simulink model "Teleoperation_no_voltage_no_force_control"  (R2020a)
settings: Solver=VariableStepAuto  StartTime=0.0  StopTime=10  RelTol=1e-3
values from neighbouring files (symbols this model uses):
  B = 1/k_m    (= 0.0517063081696)    [Teleop_parameters.m]    (also in base.mat; base_no_attrito.mat = 0; ci_siamo.mat; force_control.mat)
  Be = 5    [Teleop_parameters.m]    (also in base.mat = 0.5; base_no_attrito.mat = 0.5; ci_siamo.mat; force_control.mat = 0.5)
  Bh = 0.02    [Teleop_parameters.m]    (also in base.mat; base_no_attrito.mat; ci_siamo.mat; force_control.mat)
  Fc_h = 5    [Teleop_parameters.m]    (also in base.mat; base_no_attrito.mat; ci_siamo.mat; force_control.mat)
  J = tau_m/k_m    (= 0.0629265770424)    [Teleop_parameters.m]    (also in base.mat; base_no_attrito.mat; ci_siamo.mat; force_control.mat)
  Jh = 0.02    [Teleop_parameters.m]    (also in base.mat; base_no_attrito.mat; ci_siamo.mat; force_control.mat)
  Kd_h = 0.5    [Teleop_parameters.m]    (also in base.mat = 1; base_no_attrito.mat = 1; ci_siamo.mat = 10; force_control.mat = 1)
  Kd_m = 0.005    [Teleop_parameters.m]    (also in base.mat = 1; base_no_attrito.mat = 1; ci_siamo.mat; force_control.mat = 1)
  Kd_s = 0.5    [Teleop_parameters.m]    (also in base.mat = 1; base_no_attrito.mat = 1; ci_siamo.mat; force_control.mat = 1)
  Ke = 10    [Teleop_parameters.m]    (also in base.mat; base_no_attrito.mat; ci_siamo.mat; force_control.mat)
  Kp_h = 1.2    [Teleop_parameters.m]    (also in base.mat; base_no_attrito.mat; ci_siamo.mat = 10; force_control.mat)
  Kp_m = 0.01    [Teleop_parameters.m]    (also in base.mat = 1; base_no_attrito.mat = 1; ci_siamo.mat; force_control.mat = 1)
  Kp_s = 1    [Teleop_parameters.m]    (also in base.mat; base_no_attrito.mat; ci_siamo.mat; force_control.mat)
  qe = 1.2    [Teleop_parameters.m]    (also in base.mat = 5; base_no_attrito.mat = 5; ci_siamo.mat = 0.5; force_control.mat = 5)
settings Model: Creator=kriato  LastModifiedBy=giovanni

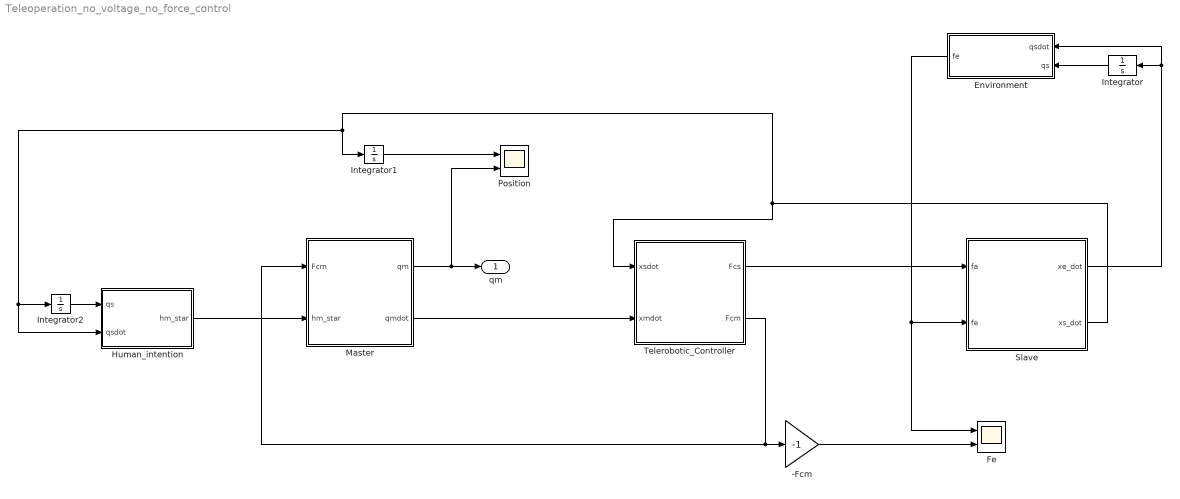
== system Teleoperation_no_voltage_no_force_control ==
  -Fcm : Gain  Gain=-1
  Environment : Subsystem
  Fe : Scope  NumInputPorts=2
  Human_intention : Subsystem
  Integrator : Integrator
  Integrator1 : Integrator
  Integrator2 : Integrator
  Master : Subsystem
  Position : Scope  NumInputPorts=2
  Slave : Subsystem
  Telerobotic_Controller : Subsystem
  qm : Outport
  wires:
  Master/2(qmdot) -> Telerobotic_Controller/2(xmdot)
  Slave/2(xs_dot) -> Human_intention/2(qsdot), Integrator2/1, Integrator1/1, Telerobotic_Controller/1(xsdot)
  Environment/1(fe) -> Slave/2(fe), Fe/1
  Master/1(qm) -> Position/2, qm/1
  Slave/1(xe_dot) -> Environment/1(qsdot), Integrator/1
  -Fcm/1 -> Fe/2
  Human_intention/1(hm_star) -> Master/2(hm_star)
  Telerobotic_Controller/1(Fcs) -> Slave/1(fa)
  Integrator/1 -> Environment/2(qs)
  Telerobotic_Controller/2(Fcm) -> Master/1(Fcm), -Fcm/1
  Integrator1/1 -> Position/1
  Integrator2/1 -> Human_intention/1(qs)

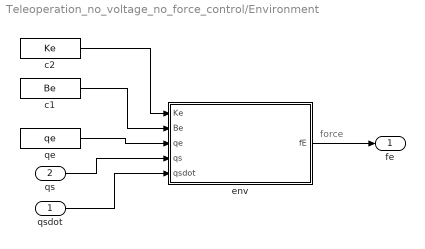
== system Teleoperation_no_voltage_no_force_control/Environment ==
  note: force
  qsdot : Inport
  qs : Inport  Port=2
  c1 : Constant  Value=Be  SampleTime=0
  c2 : Constant  Value=Ke  SampleTime=0
  env : MATLAB Function  TreatAsAtomicUnit=on
  qe : Constant  Value=qe  SampleTime=0
  fe : Outport  VectorParamsAs1DForOutWhenUnconnected=off
  wires:
  qe/1 -> env/3(qe)
  c1/1 -> env/2(Be)
  c2/1 -> env/1(Ke)
  qs/1 -> env/4(qs)
  qsdot/1 -> env/5(qsdot)
  env/1(fE) -> fe/1

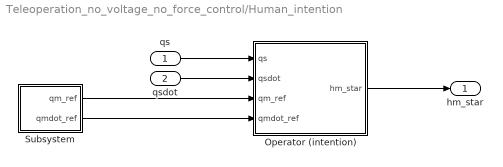
== system Teleoperation_no_voltage_no_force_control/Human_intention ==
  qs : Inport
  qsdot : Inport  Port=2
  Operator (intention) : Subsystem
  Subsystem : Subsystem
  hm_star : Outport
  wires:
  Subsystem/1(qm_ref) -> Operator (intention)/3(qm_ref)
  Subsystem/2(qmdot_ref) -> Operator (intention)/4(qmdot_ref)
  Operator (intention)/1(hm_star) -> hm_star/1
  qs/1 -> Operator (intention)/1(qs)
  qsdot/1 -> Operator (intention)/2(qsdot)

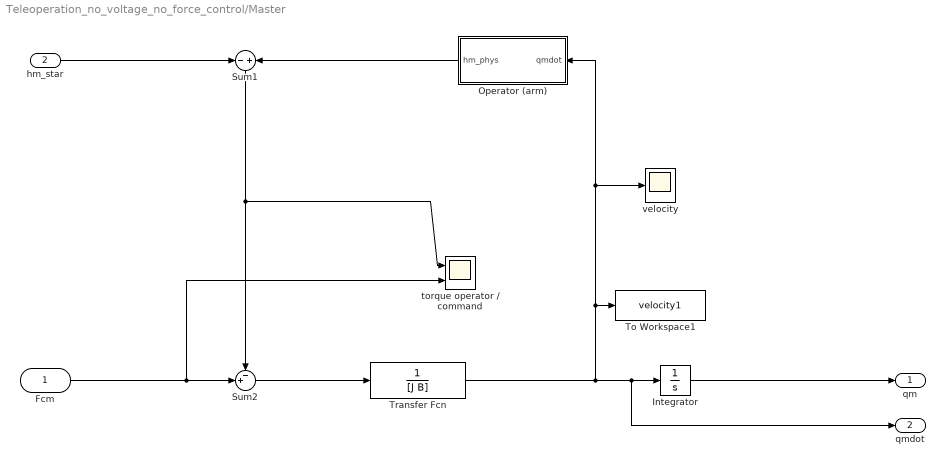
== system Teleoperation_no_voltage_no_force_control/Master ==
  Fcm : Inport
  hm_star : Inport  Port=2
  Integrator : Integrator
  Operator (arm) : Subsystem
  Sum1 : Sum  Inputs=-+
  Sum2 : Sum  Inputs=-+|
  To Workspace1 : ToWorkspace  VariableName=velocity1  SaveFormat=Timeseries  SampleTime=-1
  Transfer Fcn : TransferFcn  Denominator=[J B]
  torque operator / command : Scope  NumInputPorts=2
  velocity : Scope
  qm : Outport
  qmdot : Outport  Port=2
  wires:
  Integrator/1 -> qm/1
  Operator (arm)/1(hm_phys) -> Sum1/2
  Sum1/1 -> Sum2/1, torque operator / command/1
  Fcm/1 -> torque operator / command/2, Sum2/2
  Transfer Fcn/1 -> Operator (arm)/1(qmdot), velocity/1, To Workspace1/1, qmdot/1, Integrator/1
  hm_star/1 -> Sum1/1
  Sum2/1 -> Transfer Fcn/1

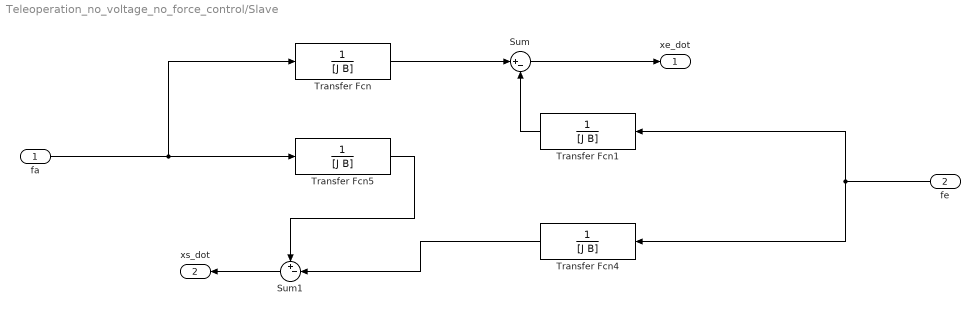
== system Teleoperation_no_voltage_no_force_control/Slave ==
  fa : Inport
  fe : Inport  Port=2
  Sum : Sum  Inputs=|+-
  Sum1 : Sum  Inputs=+-|
  Transfer Fcn{,1,4..5} (4 alike) : TransferFcn  Denominator=[J B]
  xe_dot : Outport
  xs_dot : Outport  Port=2
  wires:
  fa/1 -> Transfer Fcn5/1, Transfer Fcn/1
  Transfer Fcn/1 -> Sum/1
  Sum/1 -> xe_dot/1
  Transfer Fcn1/1 -> Sum/2
  Transfer Fcn4/1 -> Sum1/2
  Transfer Fcn5/1 -> Sum1/1
  Sum1/1 -> xs_dot/1
  fe/1 -> Transfer Fcn4/1, Transfer Fcn1/1

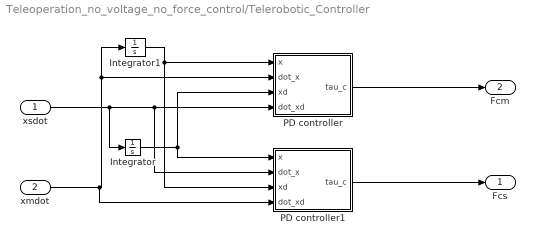
== system Teleoperation_no_voltage_no_force_control/Telerobotic_Controller ==
  xsdot : Inport
  xmdot : Inport  Port=2
  Integrator : Integrator
  Integrator1 : Integrator
  PD controller : Subsystem
  PD controller1 : Subsystem
  Fcs : Outport
  Fcm : Outport  Port=2
  wires:
  Integrator/1 -> PD controller1/1(x), PD controller/3(xd)
  Integrator1/1 -> PD controller1/3(xd), PD controller/1(x)
  xsdot/1 -> PD controller1/2(dot_x), PD controller/4(dot_xd), Integrator/1
  xmdot/1 -> PD controller1/4(dot_xd), PD controller/2(dot_x), Integrator1/1
  PD controller/1(tau_c) -> Fcm/1
  PD controller1/1(tau_c) -> Fcs/1

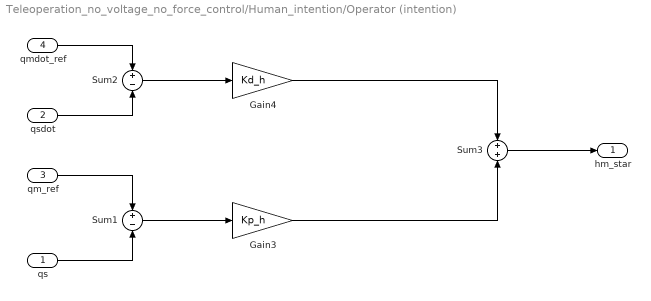
== system Teleoperation_no_voltage_no_force_control/Human_intention/Operator (intention) ==
  qs : Inport
  qsdot : Inport  Port=2
  qm_ref : Inport  Port=3
  qmdot_ref : Inport  Port=4
  Gain3 : Gain  Gain=Kp_h
  Gain4 : Gain  Gain=Kd_h
  Sum1 : Sum  Inputs=+|-
  Sum2 : Sum  Inputs=+|-
  Sum3 : Sum  Inputs=+|+
  hm_star : Outport  VectorParamsAs1DForOutWhenUnconnected=off
  wires:
  qs/1 -> Sum1/2
  qm_ref/1 -> Sum1/1
  qmdot_ref/1 -> Sum2/1
  Sum1/1 -> Gain3/1
  qsdot/1 -> Sum2/2
  Sum2/1 -> Gain4/1
  Gain4/1 -> Sum3/1
  Gain3/1 -> Sum3/2
  Sum3/1 -> hm_star/1

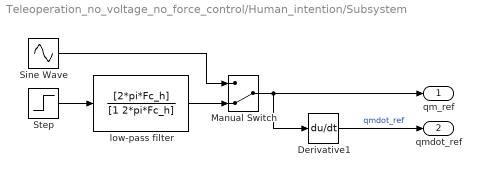
== system Teleoperation_no_voltage_no_force_control/Human_intention/Subsystem ==
  Derivative1 : Derivative  CoefficientInTFapproximation=0.001
  Manual Switch : ManualSwitch  CurrentSetting=0
  Sine Wave : Sin  SampleTime=0
  Step : Step  SampleTime=0
  low-pass filter : TransferFcn  Numerator=[2*pi*Fc_h]  Denominator=[1 2*pi*Fc_h]
  qm_ref : Outport
  qmdot_ref : Outport  Port=2
  wires:
  low-pass filter/1 -> Manual Switch/2
  Manual Switch/1 -> qm_ref/1, Derivative1/1
  Derivative1/1 -> qmdot_ref/1  "qmdot_ref"
  Step/1 -> low-pass filter/1
  Sine Wave/1 -> Manual Switch/1

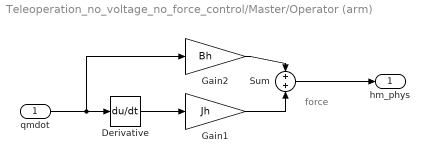
== system Teleoperation_no_voltage_no_force_control/Master/Operator (arm) ==
  note: force
  qmdot : Inport
  Derivative : Derivative  CoefficientInTFapproximation=0.001
  Gain1 : Gain  Gain=Jh
  Gain2 : Gain  Gain=Bh
  Sum : Sum  Inputs=+|+
  hm_phys : Outport  VectorParamsAs1DForOutWhenUnconnected=off
  wires:
  qmdot/1 -> Gain2/1, Derivative/1
  Sum/1 -> hm_phys/1
  Derivative/1 -> Gain1/1
  Gain2/1 -> Sum/1
  Gain1/1 -> Sum/2

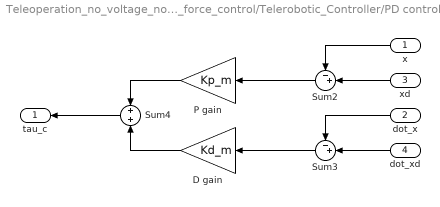
== system Teleoperation_no_voltage_no_force_control/Telerobotic_Controller/PD controller ==
  x : Inport
  dot_x : Inport  Port=2
  xd : Inport  Port=3
  dot_xd : Inport  Port=4
  D gain : Gain  Gain=Kd_m
  P gain : Gain  Gain=Kp_m
  Sum2 : Sum  Inputs=-+|
  Sum3 : Sum  Inputs=-+|
  Sum4 : Sum
  tau_c : Outport  VectorParamsAs1DForOutWhenUnconnected=off
  wires:
  D gain/1 -> Sum4/2
  dot_x/1 -> Sum3/1
  dot_xd/1 -> Sum3/2
  x/1 -> Sum2/1
  xd/1 -> Sum2/2
  Sum3/1 -> D gain/1
  P gain/1 -> Sum4/1
  Sum4/1 -> tau_c/1
  Sum2/1 -> P gain/1

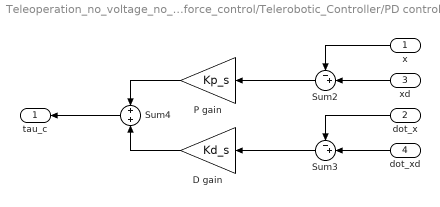
== system Teleoperation_no_voltage_no_force_control/Telerobotic_Controller/PD controller1 ==
  x : Inport
  dot_x : Inport  Port=2
  xd : Inport  Port=3
  dot_xd : Inport  Port=4
  D gain : Gain  Gain=Kd_s
  P gain : Gain  Gain=Kp_s
  Sum2 : Sum  Inputs=-+|
  Sum3 : Sum  Inputs=-+|
  Sum4 : Sum
  tau_c : Outport  VectorParamsAs1DForOutWhenUnconnected=off
  wires:
  D gain/1 -> Sum4/2
  dot_x/1 -> Sum3/1
  dot_xd/1 -> Sum3/2
  x/1 -> Sum2/1
  xd/1 -> Sum2/2
  Sum3/1 -> D gain/1
  P gain/1 -> Sum4/1
  Sum4/1 -> tau_c/1
  Sum2/1 -> P gain/1

== matlab function Teleoperation_no_voltage_no_force_control/Environment/env ==
  data: Ke input; Be input; qe input; qs input; fE output; qsdot input
function fE  = environment(Ke, Be, qe, qs, qsdot)
if qs > qe
   fE = Ke * (qs - qe) + Be * qsdot;
else
   fE = 0;
end
